simulink model "three_phase_grid_vsi_lcl"  (R2026a)
settings: Solver=ode23t  StopTime=p.sim.tStop  MaxStep=p.sim.maxStep  RelTol=0.0001  AbsTol=1e-06
InitFcn:
  | modelDir = fileparts(get_param(bdroot,'FileName'));projectDir = fileparts(modelDir);scriptDir = fullfile(projectDir,'scripts');addpath(scriptDir);run(fullfile(scriptDir,'inv_params_init.m'));run(fullfile(scriptDir,'design_lcl_filter.m'));run(fullfile(scriptDir,'tune_dq_pll_controllers.m'));
libraries: ee_lib x12, nesl_utility x11, fl_lib x1
settings Model: Creator=zheng  LastModifiedBy=zheng
settings SimscapeCC: SimscapeLogType=none

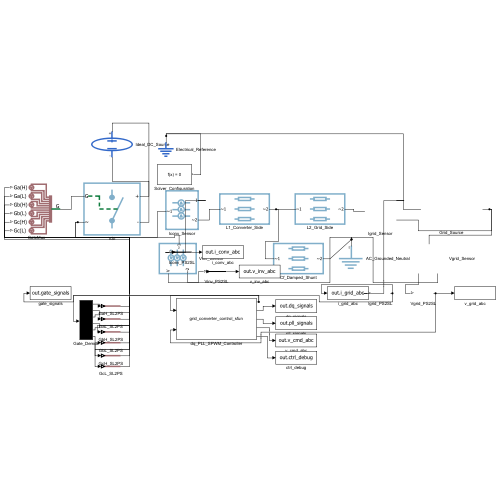
[thumbnail: Simulink's stored preview of the top-level diagram]
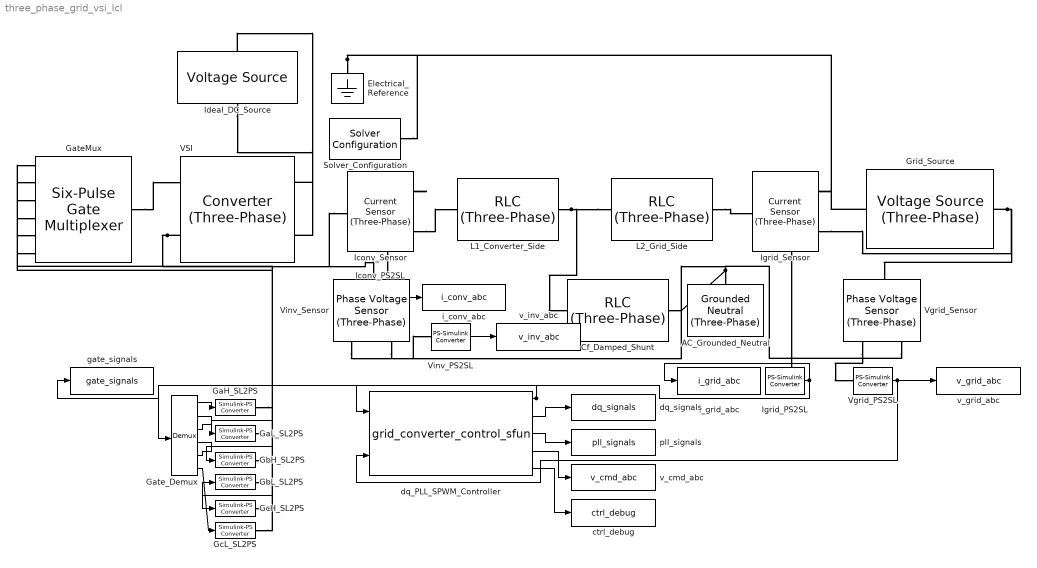
== system three_phase_grid_vsi_lcl ==
  AC_Grounded_Neutral : ee_lib/Connectors & References/Grounded Neutral (Three-Phase)  port_option=ee.enum.threePhasePort.composite
  Cf_Damped_Shunt : ee_lib/Passive/RLC Assemblies/RLC (Three-Phase)  port_option=ee.enum.threePhasePort.composite  component_structure=ee.enum.rlc.structure.SeriesRC  R=2.7217 Ohm  L=1e-3 H  C=1e-05 F  R_parasitic=0 Ohm  G_parasitic=0 1/Ohm  IL_specify=off  IL_priority=High  IL=[0, 0, 0] A  IL_nominal_specify=off  IL_nominal_value=1  IL_nominal_unit=A  VC_specify=off  VC_priority=High  VC=[0, 0, 0] V  VC_nominal_specify=off  VC_nominal_value=1  VC_nominal_unit=V
  Electrical_Reference : fl_lib/Electrical/Electrical Elements/Electrical Reference
  GaH_SL2PS : nesl_utility/Simulink-PS Converter  PhysicalDomain=network_engine_domain  SubClassName=ps_input  LeftPortType=input  RightPortType=output  PseudoPeriodic=off  Frequencies=[]  NoiseDistribution=none  NoiseParameters=[]  Unit=V  AffineConversion=off  FilteringAndDerivatives=zero  SimscapeFilterOrder=1  InputFilterTimeConstant=0.001  UdotUserProvided=0
  GaL_SL2PS : nesl_utility/Simulink-PS Converter  PhysicalDomain=network_engine_domain  SubClassName=ps_input  LeftPortType=input  RightPortType=output  PseudoPeriodic=off  Frequencies=[]  NoiseDistribution=none  NoiseParameters=[]  Unit=V  AffineConversion=off  FilteringAndDerivatives=zero  SimscapeFilterOrder=1  InputFilterTimeConstant=0.001  UdotUserProvided=0
  GateMux : ee_lib/Semiconductors & Converters/Converters/Six-Pulse Gate Multiplexer  port_option=ee.enum.controlport.ps
  Gate_Demux : Demux  Outputs=6
  GbH_SL2PS : nesl_utility/Simulink-PS Converter  PhysicalDomain=network_engine_domain  SubClassName=ps_input  LeftPortType=input  RightPortType=output  PseudoPeriodic=off  Frequencies=[]  NoiseDistribution=none  NoiseParameters=[]  Unit=V  AffineConversion=off  FilteringAndDerivatives=zero  SimscapeFilterOrder=1  InputFilterTimeConstant=0.001  UdotUserProvided=0
  GbL_SL2PS : nesl_utility/Simulink-PS Converter  PhysicalDomain=network_engine_domain  SubClassName=ps_input  LeftPortType=input  RightPortType=output  PseudoPeriodic=off  Frequencies=[]  NoiseDistribution=none  NoiseParameters=[]  Unit=V  AffineConversion=off  FilteringAndDerivatives=zero  SimscapeFilterOrder=1  InputFilterTimeConstant=0.001  UdotUserProvided=0
  GcH_SL2PS : nesl_utility/Simulink-PS Converter  PhysicalDomain=network_engine_domain  SubClassName=ps_input  LeftPortType=input  RightPortType=output  PseudoPeriodic=off  Frequencies=[]  NoiseDistribution=none  NoiseParameters=[]  Unit=V  AffineConversion=off  FilteringAndDerivatives=zero  SimscapeFilterOrder=1  InputFilterTimeConstant=0.001  UdotUserProvided=0
  GcL_SL2PS : nesl_utility/Simulink-PS Converter  PhysicalDomain=network_engine_domain  SubClassName=ps_input  LeftPortType=input  RightPortType=output  PseudoPeriodic=off  Frequencies=[]  NoiseDistribution=none  NoiseParameters=[]  Unit=V  AffineConversion=off  FilteringAndDerivatives=zero  SimscapeFilterOrder=1  InputFilterTimeConstant=0.001  UdotUserProvided=0
  Grid_Source : ee_lib/Sources/Voltage Source (Three-Phase)  vline_rms=293.938769134 V  shift=0 deg  freq=50 Hz  impedance_option=1  SShortCircuit=100e6 A*V  XR=10  R=0.01 Ohm  L=3.97e-4 H  harmonic_option=0  harmonic_orders=[5, 7, 11, 13]  harmonic_ratios=[.1, .1, .1, .1]  G_parasitic=0 1/Ohm  I_specify=off  I_priority=None  I=[0, 0, 0] A  I_nominal_specify=off  I_nominal_value=1  I_nominal_unit=A
  Iconv_PS2SL : nesl_utility/PS-Simulink Converter  PhysicalDomain=network_engine_domain  SubClassName=ps_output  LeftPortType=input  RightPortType=output  PseudoPeriodic=off  Frequencies=[]  VectorFormat=1-D array  Unit=A  AffineConversion=off
  Iconv_Sensor : ee_lib/Sensors & Transducers/Current Sensor (Three-Phase)  port_option=ee.enum.threePhasePort.composite
  Ideal_DC_Source : ee_lib/Sources/Voltage Source  dc_voltage=800 V  ac_voltage=0 V  ac_shift=0 rad  ac_frequency=60 Hz  noise_mode=ee.enum.sources.noise.Disabled  PSD=0 V^2/Hz  sample_time=1e-3 s  repeatability=ee.enum.sources.repeatability.NotRepeatable  user_seed=0  auto_seed=4112460543  i_specify=off  i_priority=None  i=0 A  i_nominal_specify=off  i_nominal_value=1  i_nominal_unit=A  v_specify=off  v_priority=None  v=0 V  v_nominal_specify=off  v_nominal_value=1  v_nominal_unit=V
  Igrid_PS2SL : nesl_utility/PS-Simulink Converter  PhysicalDomain=network_engine_domain  SubClassName=ps_output  LeftPortType=input  RightPortType=output  PseudoPeriodic=off  Frequencies=[]  VectorFormat=1-D array  Unit=A  AffineConversion=off
  Igrid_Sensor : ee_lib/Sensors & Transducers/Current Sensor (Three-Phase)  port_option=ee.enum.threePhasePort.composite
  L1_Converter_Side : ee_lib/Passive/RLC Assemblies/RLC (Three-Phase)  port_option=ee.enum.threePhasePort.composite  component_structure=ee.enum.rlc.structure.SeriesRL  R=0.05 Ohm  L=0.002 H  C=1e-6 F  R_parasitic=0 Ohm  G_parasitic=0 1/Ohm  IL_specify=off  IL_priority=High  IL=[0, 0, 0] A  IL_nominal_specify=off  IL_nominal_value=1  IL_nominal_unit=A  VC_specify=off  VC_priority=High  VC=[0, 0, 0] V  VC_nominal_specify=off  VC_nominal_value=1  VC_nominal_unit=V
  L2_Grid_Side : ee_lib/Passive/RLC Assemblies/RLC (Three-Phase)  port_option=ee.enum.threePhasePort.composite  component_structure=ee.enum.rlc.structure.SeriesRL  R=0.05 Ohm  L=0.001 H  C=1e-6 F  R_parasitic=0 Ohm  G_parasitic=0 1/Ohm  IL_specify=off  IL_priority=High  IL=[0, 0, 0] A  IL_nominal_specify=off  IL_nominal_value=1  IL_nominal_unit=A  VC_specify=off  VC_priority=High  VC=[0, 0, 0] V  VC_nominal_specify=off  VC_nominal_value=1  VC_nominal_unit=V
  Solver_Configuration : nesl_utility/Solver Configuration  PhysicalDomain=network_engine_domain  SubClassName=solver  LeftPortType=input  RightPortType=generic  Tones=[]  Harmonics=[]  SimulateNoise=off  Profile=off  UseLocalSampling=off  EnableSwitchedLinearOptims=on  FrequencyDomain=off  UseCCode=off  RelTol=0.001  AbsTol=0.001  MinStep=1e-09  ToWorkspace=off  RevertToSquareIcSolve=off  NumHomotopyIterations=100  PhasorMode=off  PhasorModeNumHarmonics=1  ConsistencySolver=NEWTON_XTOL_AFTER_FTOL  CanonicalOrdering=CANONICAL  OptimizeIntermediates=OPTIMIZED  IndexReductionMethod=DerivativeReplacement  DoDC=off  ResidualTolerance=1e-09  ConsistencyTolSource=GLOBAL  ConsistencyAbsTol=0.001  ConsistencyRelTol=0.001  ConsistencyTolFactor=0.001  UseLocalSolver=off  LocalSolverChoice=NE_BACKWARD_EULER_ADVANCER  ResolveIndetEquations=on  FunctionEvalNumThread=1  LocalSolverSampleTime=0.001  DoFixedCost=off  MaxNonlinIter=3  MaxModeIter=2  ComputeImpulses=off  ImpulseIterations=2  LinearAlgebra=auto  LinearAlgebraNumThread=0  EquationFormulation=NE_TIME_EF  DelaysMemoryBudget=1024  AutomaticFiltering=on  FilteringTimeConstant=0.001  PartitionStorageMethod=AS_NEEDED  PartitionMemoryBudget=1024  PartitionMethod=ROBUST  MultibodyUseLocalSolver=off  MultibodyLocalSolverChoice=ODE1  MultibodyLocalSolverSampleTime=0.001
  VSI : ee_lib/Semiconductors & Converters/Converters/Converter (Three-Phase)  port_option=ee.enum.threePhasePort.composite  fidelity_option=ee.enum.converters.fidelity.detailed  device_type=ee.enum.converters.switchingdevice.ideal  showThermalPort=false  K=0  Vth=6 V  Vgt=6 V  Vgt_off=-1 V  Ih=1 A  Vf=0.8 V  Ron=0.001 Ohm  Rds=0.001 Ohm  Goff=1e-06 1/Ohm  Eon_scalar=22.86e-3 J  Eoff_scalar=17.14e-3 J  Eoff_natural_commutation=10e-3 J  Voff=300 V  Iout_scalar=600 A  onCurrentMeasDelay=0 s  useCurrentFromPreviousCycle=false  useVoltageFromPreviousCycle=false  diode_param=ee.enum.converters.protectiondiode.nodynamics  diode_Vf=0.8 V  diode_Ron=0.001 Ohm  diode_Goff=1e-06 1/Ohm  diode_C=50 nF  diode_iRM=-235 A  diode_iF=300 A  diode_idot=-50 A/us  diode_trr_param=ee.enum.converters.diodetrr.trr_factor  diode_trr_factor=3  diode_trr=15 us  diode_Qrr=1500 s*uA  diode_rec_loss_model=ee.enum.diode.reverseRecoveryModel.fixed  diode_ErecVal=0 J  diode_scaleWithIandV=false  diode_ErecMat=zeros(2, 3) J  diode_TjrecVec=[298.15, 398.15] K  diode_IfrecVec=[.1, 1, 10] A  diode_IrecVal=10 A  diode_VrecVal=10 V  diode_tFilter=1 / 1000 / 100 s  thermal_network_parameterization=ee.enum.thermalNetworkTopology.external  Rth=[.08, .5] K/W  Rth_Cauer=[.08, .1, .5] K/W  Rth_Foster=[.08, .14, .22, .16] K/W  thermal_mass_parameterization=ee.enum.thermalNetwork.timeconstant  thermal_mass=[.01, .5] J/K  thermal_mass_Cauer=[.01, .1, .5] J/K  thermal_mass_Foster=[.001, .005, .05, .5] J/K  thermal_time_constant=[.001, .2] s  thermal_time_constant_Cauer=[.001, .1, .2] s  thermal_time_constant_Foster=[7e-05, .0007, .01, .08] s  thermal_mass_initial_temperatures=[25, 25] degC  thermal_mass_initial_temperatures_Cauer=[25, 25, 25] degC  junction_thermal_mass=0.01 J/K  Tvec_initial_Foster=[25, 25, 25, 25] degC  snubber_type=ee.enum.converters.snubber.exclude  Cs=1e-7 F  Rs=0.1 Ohm  Vce_loss=[0, 150, 300] V
  Vgrid_PS2SL : nesl_utility/PS-Simulink Converter  PhysicalDomain=network_engine_domain  SubClassName=ps_output  LeftPortType=input  RightPortType=output  PseudoPeriodic=off  Frequencies=[]  VectorFormat=1-D array  Unit=V  AffineConversion=off
  Vgrid_Sensor : ee_lib/Sensors & Transducers/Phase Voltage Sensor (Three-Phase)  port_option=ee.enum.threePhasePort.composite
  Vinv_PS2SL : nesl_utility/PS-Simulink Converter  PhysicalDomain=network_engine_domain  SubClassName=ps_output  LeftPortType=input  RightPortType=output  PseudoPeriodic=off  Frequencies=[]  VectorFormat=1-D array  Unit=V  AffineConversion=off
  Vinv_Sensor : ee_lib/Sensors & Transducers/Phase Voltage Sensor (Three-Phase)  port_option=ee.enum.threePhasePort.composite
  ctrl_debug : ToWorkspace  VariableName=ctrl_debug  SaveFormat=Timeseries  SampleTime=-1
  dq_PLL_SPWM_Controller : M-S-Function  FunctionName=grid_converter_control_sfun  Parameters=p
  dq_signals : ToWorkspace  VariableName=dq_signals  SaveFormat=Timeseries  SampleTime=-1
  gate_signals : ToWorkspace  VariableName=gate_signals  SaveFormat=Timeseries  SampleTime=-1
  i_conv_abc : ToWorkspace  VariableName=i_conv_abc  SaveFormat=Timeseries  SampleTime=-1
  i_grid_abc : ToWorkspace  VariableName=i_grid_abc  SaveFormat=Timeseries  SampleTime=-1
  pll_signals : ToWorkspace  VariableName=pll_signals  SaveFormat=Timeseries  SampleTime=-1
  v_cmd_abc : ToWorkspace  VariableName=v_cmd_abc  SaveFormat=Timeseries  SampleTime=-1
  v_grid_abc : ToWorkspace  VariableName=v_grid_abc  SaveFormat=Timeseries  SampleTime=-1
  v_inv_abc : ToWorkspace  VariableName=v_inv_abc  SaveFormat=Timeseries  SampleTime=-1
  wires:
  Igrid_PS2SL/1 -> dq_PLL_SPWM_Controller/1, i_grid_abc/1
  Vgrid_PS2SL/1 -> dq_PLL_SPWM_Controller/2, v_grid_abc/1
  dq_PLL_SPWM_Controller/1 -> Gate_Demux/1, gate_signals/1
  dq_PLL_SPWM_Controller/2 -> dq_signals/1
  dq_PLL_SPWM_Controller/3 -> pll_signals/1
  dq_PLL_SPWM_Controller/4 -> v_cmd_abc/1
  dq_PLL_SPWM_Controller/5 -> ctrl_debug/1
  Iconv_PS2SL/1 -> i_conv_abc/1
  Vinv_PS2SL/1 -> v_inv_abc/1
  Gate_Demux/1 -> GaH_SL2PS/1
  Gate_Demux/2 -> GaL_SL2PS/1
  Gate_Demux/3 -> GbH_SL2PS/1
  Gate_Demux/4 -> GbL_SL2PS/1
  Gate_Demux/5 -> GcH_SL2PS/1
  Gate_Demux/6 -> GcL_SL2PS/1
  connections:
  Ideal_DC_Source/LConn1 -- VSI/RConn1
  Ideal_DC_Source/RConn1 -- VSI/RConn2
  Electrical_Reference/LConn1 -- Grid_Source/LConn1 -- Solver_Configuration/RConn1
  GateMux/RConn1 -- VSI/LConn1
  Iconv_Sensor/LConn1 -- VSI/LConn2 -- Vinv_Sensor/LConn1
  Vinv_Sensor/RConn2 -- Cf_Damped_Shunt/RConn1 -- AC_Grounded_Neutral/LConn1 -- Vgrid_Sensor/RConn2
  Iconv_Sensor/RConn2 -- L1_Converter_Side/LConn1
  L2_Grid_Side/LConn1 -- L1_Converter_Side/RConn1 -- Cf_Damped_Shunt/LConn1
  L2_Grid_Side/RConn1 -- Igrid_Sensor/LConn1
  Grid_Source/RConn1 -- Igrid_Sensor/RConn2 -- Vgrid_Sensor/LConn1
  Iconv_Sensor/RConn1 -- Iconv_PS2SL/LConn1
  Vinv_Sensor/RConn1 -- Vinv_PS2SL/LConn1
  Igrid_Sensor/RConn1 -- Igrid_PS2SL/LConn1
  Vgrid_Sensor/RConn1 -- Vgrid_PS2SL/LConn1
  GaH_SL2PS/RConn1 -- GateMux/LConn1
  GaL_SL2PS/RConn1 -- GateMux/LConn2
  GbH_SL2PS/RConn1 -- GateMux/LConn3
  GbL_SL2PS/RConn1 -- GateMux/LConn4
  GcH_SL2PS/RConn1 -- GateMux/LConn5
  GcL_SL2PS/RConn1 -- GateMux/LConn6
